simulink model "sim_sliding"  (R2015a)
settings: Solver=ode4  StartTime=0.0  StopTime=150  FixedStep=0.005  RelTol=1e-3
undefined symbols (not defined in the file or in its folder): C11a, G21a, M11, M21a, M21b, M22, rk, rw
settings Model: CovSFcnEnable=off  Creator=desti  LastModifiedBy=desti
settings DebuggingCC: SolverPrmCheckMsg=warning

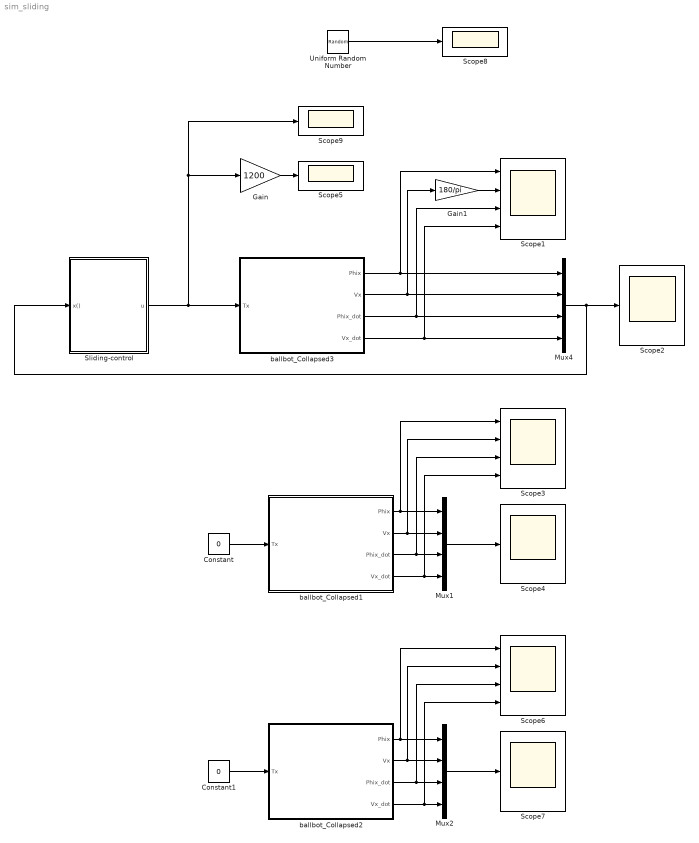
== system sim_sliding ==
  Constant : Constant  Value=0
  Constant1 : Constant  Value=0
  Gain : Gain  Gain=1200
  Gain1 : Gain  Gain=180/pi
  Mux1 : Mux
  Mux2 : Mux
  Mux4 : Mux
  Scope1 : Scope  NumInputPorts=4
      settings: TimeRange=1  YMin=0~-5~-5~-5  YMax=1~5~5~5  SaveName=Vx
  Scope{2,4..5,7..9} (6 alike) : Scope
      Scope2 settings: TimeRange=1  YMin=0  YMax=1  SaveName=Vx2
      Scope4 settings: TimeRange=1  YMin=0  YMax=1  SaveName=Vx3
      Scope5 settings: TimeRange=1  YMin=0  YMax=1  SaveName=Vx4
      Scope7 settings: TimeRange=1  YMin=0  YMax=1  SaveName=Vx6
      Scope8 settings: TimeRange=1  YMin=0  YMax=1  SaveName=Vx7
      Scope9 settings: TimeRange=1  YMin=0  YMax=1  SaveName=Vx8
  Scope3 : Scope  NumInputPorts=4
      settings: TimeRange=1  YMin=0~-5~-5~-5  YMax=1~5~5~5  SaveName=Vx1
  Scope6 : Scope  NumInputPorts=4
      settings: TimeRange=1  YMin=0~-5~-5~-5  YMax=1~5~5~5  SaveName=Vx5
  Sliding-control : Subsystem
  Uniform Random Number : UniformRandomNumber  Minimum=-2*pi/180  Maximum=2*pi/180  Seed=100  SampleTime=0.005
  ballbot_Collapsed1 : Subsystem
  ballbot_Collapsed2 : Subsystem
  ballbot_Collapsed3 : Subsystem
  wires:
  Mux4/1 -> Sliding-control/1(x()), Scope2/1
  ballbot_Collapsed3/4(Vx_dot) -> Scope1/4, Mux4/4
  ballbot_Collapsed3/3(Phix_dot) -> Scope1/3, Mux4/3
  ballbot_Collapsed3/2(Vx) -> Gain1/1, Mux4/2
  ballbot_Collapsed3/1(Phix) -> Scope1/1, Mux4/1
  Sliding-control/1(u) -> ballbot_Collapsed3/1(Tx), Scope9/1, Gain/1
  Mux1/1 -> Scope4/1
  ballbot_Collapsed1/4(Vx_dot) -> Mux1/4, Scope3/4
  ballbot_Collapsed1/3(Phix_dot) -> Mux1/3, Scope3/3
  ballbot_Collapsed1/2(Vx) -> Mux1/2, Scope3/2
  ballbot_Collapsed1/1(Phix) -> Mux1/1, Scope3/1
  Constant/1 -> ballbot_Collapsed1/1(Tx)
  Mux2/1 -> Scope7/1
  ballbot_Collapsed2/4(Vx_dot) -> Scope6/4, Mux2/4
  ballbot_Collapsed2/3(Phix_dot) -> Scope6/3, Mux2/3
  ballbot_Collapsed2/2(Vx) -> Scope6/2, Mux2/2
  ballbot_Collapsed2/1(Phix) -> Scope6/1, Mux2/1
  Constant1/1 -> ballbot_Collapsed2/1(Tx)
  Gain/1 -> Scope5/1
  Uniform Random Number/1 -> Scope8/1
  Gain1/1 -> Scope1/2

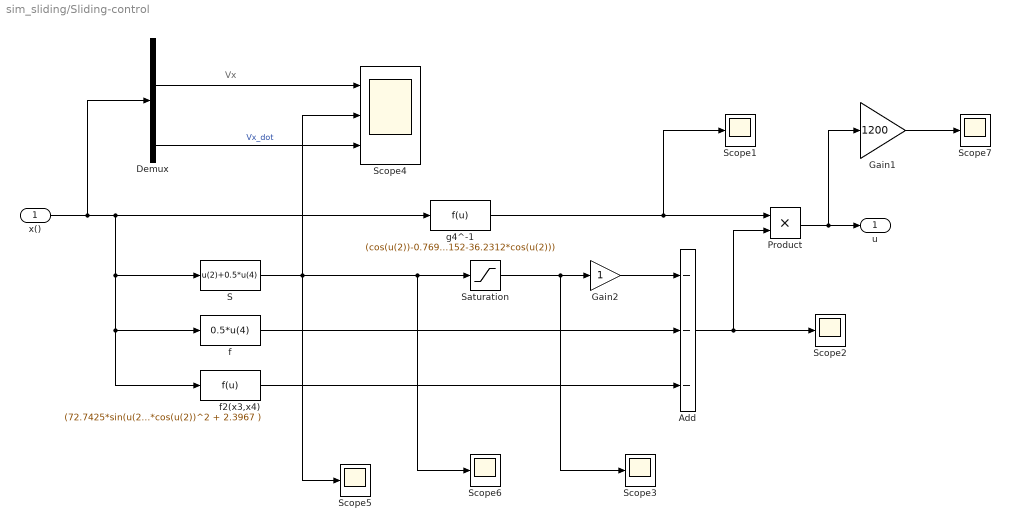
== system sim_sliding/Sliding-control ==
  note: Vx
  x() : Inport
  Add : Sum  Inputs=---
  Demux : Demux
  Gain1 : Gain  Gain=1200
  Gain2 : Gain
  Product : Product
  S : Fcn  Expr=u(2)+0.5*u(4)
  Saturation : Saturate  UpperLimit=0.2  LowerLimit=-0.2
  Scope{1..3,5..7} (6 alike) : Scope
      Scope2 settings: SaveName=ScopeData2
      Scope3 settings: SaveName=ScopeData3
      Scope6 settings: SaveName=ScopeData5
      Scope7 settings: SaveName=ScopeData8
  Scope4 : Scope  NumInputPorts=3
      settings: YMin=-5~-5~-5  YMax=5~5~5  SaveName=ScopeData4
  f : Fcn  Expr=0.5*u(4)
  f2(x3,x4) : Fcn  Expr=(72.7425*sin(u(2)) - 0.7693*cos(u(2))*sin(u(2))*u(4)^2 + 0.5*sin(u(2))*u(4)^2 ) / ( cos(u(2)) - 0.7693*cos(u(2))^2 + 2.3967 )
  g4^-1 : Fcn  Expr=(cos(u(2))-0.7693*(cos(u(2)))^2+2.3967) / (-19.2152-36.2312*cos(u(2)))
  u : Outport
  wires:
  g4^-1/1 -> Scope1/1, Product/1
  x()/1 -> Demux/1, g4^-1/1, S/1, f/1, f2(x3,x4)/1
  Add/1 -> Scope2/1, Product/2
  Product/1 -> Gain1/1, u/1
  Saturation/1 -> Gain2/1, Scope3/1
  f/1 -> Add/2
  f2(x3,x4)/1 -> Add/3
  S/1 -> Scope6/1, Saturation/1, Scope4/2, Scope5/1
  Gain2/1 -> Add/1
  Demux/2 -> Scope4/1
  Demux/4 -> Scope4/3  "Vx_dot"
  Gain1/1 -> Scope7/1

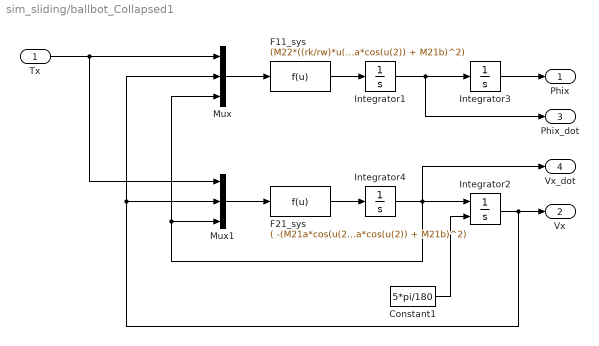
== system sim_sliding/ballbot_Collapsed1 ==
  Tx : Inport
  Constant1 : Constant  Value=5*pi/180
  F11_sys : Fcn  Expr=(M22*((rk/rw)*u(1) - C11a*sin(u(2))*(u(3))^2) + (M21a*cos(u(2)) + M21b)*((rk/rw)*u(1) + G21a*sin(u(2)))) / (M11*M22 - (M21a*cos(u(2)) + M21b)^2)
  F21_sys : Fcn  Expr=( -(M21a*cos(u(2)) + M21b)*((rk/rw)*u(1) - C11a*sin(u(2))*(u(3))^2) - M11*((rk/rw)*u(1) + G21a*sin(u(2))) ) / (M11*M22 - (M21a*cos(u(2)) + M21b)^2)
  Integrator1 : Integrator
  Integrator2 : Integrator  InitialConditionSource=external
  Integrator3 : Integrator
  Integrator4 : Integrator
  Mux : Mux  Inputs=3
  Mux1 : Mux  Inputs=3
  Phix : Outport
  Vx : Outport  Port=2
  Phix_dot : Outport  Port=3
  Vx_dot : Outport  Port=4
  wires:
  Constant1/1 -> Integrator2/2
  Tx/1 -> Mux/1, Mux1/1
  F11_sys/1 -> Integrator1/1
  Mux/1 -> F11_sys/1
  Mux1/1 -> F21_sys/1
  F21_sys/1 -> Integrator4/1
  Integrator2/1 -> Mux1/2, Mux/2, Vx/1
  Integrator3/1 -> Phix/1
  Integrator1/1 -> Phix_dot/1, Integrator3/1
  Integrator4/1 -> Mux1/3, Mux/3, Vx_dot/1, Integrator2/1

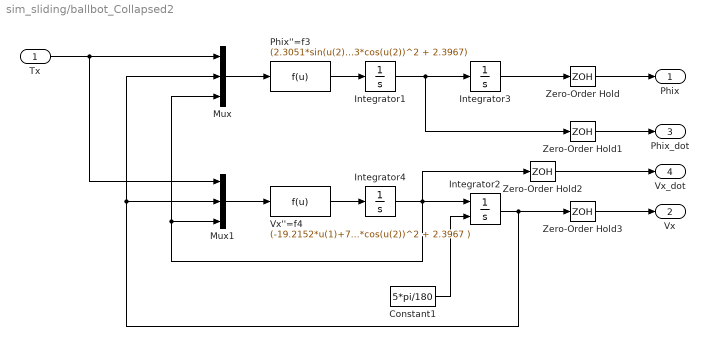
== system sim_sliding/ballbot_Collapsed2 ==
  Tx : Inport
  Constant1 : Constant  Value=5*pi/180
  Integrator1 : Integrator
  Integrator2 : Integrator  InitialConditionSource=external
  Integrator3 : Integrator
  Integrator4 : Integrator
  Mux : Mux  Inputs=3
  Mux1 : Mux  Inputs=3
  Phix''=f3 : Fcn  Expr=(2.3051*sin(u(2))*u(3)^2 + 85.0154*u(1) + 36.2312*u(1)*cos(u(2)) - 61.6090*cos(u(2))*sin(u(2)) + 40.0377*sin(u(2))) / (cos(u(2)) - 0.7693*cos(u(2))^2 + 2.3967)
  Vx''=f4 : Fcn  Expr=(-19.2152*u(1)+72.7425*sin(u(2))-0.7693*cos(u(2))*sin(u(2))*u(3)^2-36.2312*cos(u(2))*u(1)+0.5*sin(u(2))*u(3)^2) / (cos(u(2)) - 0.7693*cos(u(2))^2 + 2.3967 )
  Zero-Order Hold{,1..3} (4 alike) : ZeroOrderHold  SampleTime=0.005
  Phix : Outport
  Vx : Outport  Port=2
  Phix_dot : Outport  Port=3
  Vx_dot : Outport  Port=4
  wires:
  Zero-Order Hold3/1 -> Vx/1
  Zero-Order Hold2/1 -> Vx_dot/1
  Zero-Order Hold1/1 -> Phix_dot/1
  Zero-Order Hold/1 -> Phix/1
  Constant1/1 -> Integrator2/2
  Tx/1 -> Mux/1, Mux1/1
  Phix''=f3/1 -> Integrator1/1
  Mux/1 -> Phix''=f3/1
  Mux1/1 -> Vx''=f4/1
  Vx''=f4/1 -> Integrator4/1
  Integrator2/1 -> Mux1/2, Mux/2, Zero-Order Hold3/1
  Integrator3/1 -> Zero-Order Hold/1
  Integrator1/1 -> Zero-Order Hold1/1, Integrator3/1
  Integrator4/1 -> Mux1/3, Mux/3, Zero-Order Hold2/1, Integrator2/1

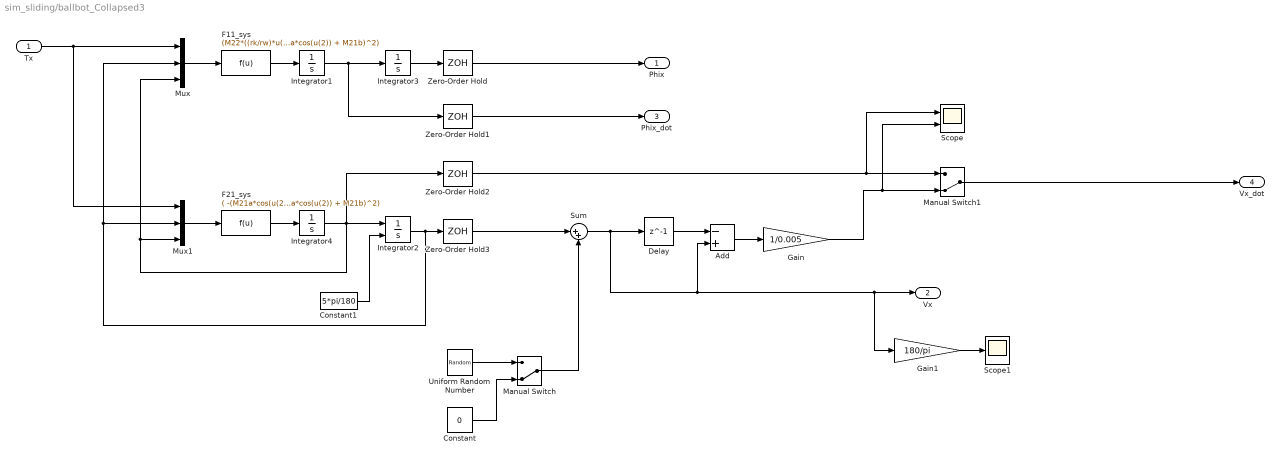
== system sim_sliding/ballbot_Collapsed3 ==
  Tx : Inport
  Add : Sum  Inputs=-+
  Constant : Constant  Value=0
  Constant1 : Constant  Value=5*pi/180
  Delay : Delay  DelayLength=1
  F11_sys : Fcn  Expr=(M22*((rk/rw)*u(1) - C11a*sin(u(2))*(u(3))^2) + (M21a*cos(u(2)) + M21b)*((rk/rw)*u(1) + G21a*sin(u(2)))) / (M11*M22 - (M21a*cos(u(2)) + M21b)^2)
  F21_sys : Fcn  Expr=( -(M21a*cos(u(2)) + M21b)*((rk/rw)*u(1) - C11a*sin(u(2))*(u(3))^2) - M11*((rk/rw)*u(1) + G21a*sin(u(2))) ) / (M11*M22 - (M21a*cos(u(2)) + M21b)^2)
  Gain : Gain  Gain=1/0.005
  Gain1 : Gain  Gain=180/pi
  Integrator1 : Integrator
  Integrator2 : Integrator  InitialConditionSource=external
  Integrator3 : Integrator
  Integrator4 : Integrator
  Manual Switch : ManualSwitch  CurrentSetting=0
  Manual Switch1 : ManualSwitch  CurrentSetting=0
  Mux : Mux  Inputs=3
  Mux1 : Mux  Inputs=3
  Scope : Scope  NumInputPorts=2
      settings: YMin=-5~-5  YMax=5~5  SaveName=ScopeData6
  Scope1 : Scope
      settings: SaveName=ScopeData7
  Sum : Sum  Inputs=|++
  Uniform Random Number : UniformRandomNumber  Minimum=-0.2*pi/180  Maximum=0.2*pi/180  SampleTime=0.005
  Zero-Order Hold{,1..3} (4 alike) : ZeroOrderHold  SampleTime=0.005
  Phix : Outport
  Vx : Outport  Port=2
  Phix_dot : Outport  Port=3
  Vx_dot : Outport  Port=4
  wires:
  Integrator4/1 -> Integrator2/1, Zero-Order Hold2/1, Mux/3, Mux1/3
  Integrator1/1 -> Integrator3/1, Zero-Order Hold1/1
  Integrator3/1 -> Zero-Order Hold/1
  Integrator2/1 -> Zero-Order Hold3/1, Mux/2, Mux1/2
  F21_sys/1 -> Integrator4/1
  Mux1/1 -> F21_sys/1
  Mux/1 -> F11_sys/1
  F11_sys/1 -> Integrator1/1
  Tx/1 -> Mux1/1, Mux/1
  Constant1/1 -> Integrator2/2
  Zero-Order Hold/1 -> Phix/1
  Zero-Order Hold1/1 -> Phix_dot/1
  Zero-Order Hold2/1 -> Scope/1, Manual Switch1/1
  Zero-Order Hold3/1 -> Sum/1
  Sum/1 -> Delay/1, Gain1/1, Vx/1, Add/2
  Delay/1 -> Add/1
  Add/1 -> Gain/1
  Gain/1 -> Scope/2, Manual Switch1/2
  Uniform Random Number/1 -> Manual Switch/1
  Constant/1 -> Manual Switch/2
  Manual Switch/1 -> Sum/2
  Manual Switch1/1 -> Vx_dot/1
  Gain1/1 -> Scope1/1
